simulink library "GOcontroll_Moduline_Target"  (R2018b)
settings: Solver=ode45  StartTime=0.0  StopTime=10.0  RelTol=1e-3  EnableMultiTasking=on
(part 3 of 3)

== system GOcontroll_Moduline_Target/Modules/Output Module ==
  Output Module (10 channel) : Subsystem  Tag=HANcoder_GOcontroll_Moduline_IV  mask(10 Channel Output Module){tsamp=0.1, ContrType=GOcontroll Moduline IV, moduleSlot=Moduleslot 1, C12freq=200 Hz, C1func=Disable (output disabled), C1peakDuty=1000, C1peakTime=500, C2func=Disable (output disabled), C2peakDuty=1000, C2peakTime=500, C34freq=200 Hz, C3func=Disable (output disabled), C3peakDuty=1000, C3peakTime=500, C4func=Disable (output disabled), C4peakDuty=1000, C4peakTime=500, C56freq=200 Hz, C5func=Disable (output disabled), C5peakDuty=1000, C5peakTime=500, C6func=Disable (output disabled), C6peakDuty=1000, C6peakTime=500, C78freq=200 Hz, C7func=Disable (output disabled), C7peakDuty=1000, C7peakTime=500, C8func=Disable (output disabled), C8peakDuty=1000, C8peakTime=500, C910freq=200 Hz, C9func=Disable (output disabled), C9peakDuty=1000, C9peakTime=500, C10func=Disable (output disabled), C10peakDuty=1000, C10peakTime=500}
      mask prompts: tsamp "Sample time"; ContrType "Controller type"; moduleSlot "Module slot"; C12freq "Frequency"; C1func "Channel 1 function"; C1peakDuty "Peak Duty-Cycle (0-1000)"; C1peakTime "Peak time (ms)"; C2func "Channel 2 function"; C2peakDuty "Peak Duty-Cycle (0-1000)"; C2peakTime "Peak time (ms)"; C34freq "Frequency"; C3func "Channel 3 function"; C3peakDuty "Peak Duty-Cycle (0-1000)"; C3peakTime "Peak time (ms)"; C4func "Channel 4 function"; C4peakDuty "Peak Duty-Cycle (0-1000)"; C4peakTime "Peak time (ms)"; C56freq "Frequency"; C5func "Channel 5 function"; C5peakDuty "Peak Duty-Cycle (0-1000)"; C5peakTime "Peak time (ms)"; C6func "Channel 6 function"; C6peakDuty "Peak Duty-Cycle (0-1000)"; C6peakTime "Peak time (ms)"; C78freq "Frequency"; C7func "Channel 7 function"; C7peakDuty "Peak Duty-Cycle (0-1000)"; C7peakTime "Peak time (ms)"; C8func "Channel 8 function"; C8peakDuty "Peak Duty-Cycle (0-1000)"; C8peakTime "Peak time (ms)"; C910freq "Frequency"; C9func "Channel 9 function"; C9peakDuty "Peak Duty-Cycle (0-1000)"; C9peakTime "Peak time (ms)"; C10func "Channel 10 function"; C10peakDuty "Peak Duty-Cycle (0-1000)"; C10peakTime "Peak time (ms)"
      mask help:
      | With this function block, you can configure each output of the 6 channel output module (202002xx). During initialization of the controller, the corresponding outputs of the module are set according the settings. During runtime, the value pushed into the block will control the outputs.
      |
      | Sample time:
      | Execution frequency from function block. For proper functioning of the output module, us a sampletime of 100 ms or lower.
      |
      | Module slot:
      | Sets the location of the module slot where the module is physically plugged into.
      |
      | Frequency:
      | In case a duty Cycle is used, select the frequency.
      |
      | Function select:
      | Select the desired output configuration for each channel
      mask init:
      | [moduleSlotInfoStr, connectorId, pin1Id, pin2Id, pin3Id, pin4Id, pin5Id, pin6Id, pin7Id, pin8Id, pin9Id, pin10Id] = sfcn_gocontroll_output_module_10_mcb(moduleSlot,ContrType,...
      | C12freq,C1func,C2func,C34freq,C3func,C4func,C56freq,C5func,C6func,C78freq,C7func,C8func,C910freq,C9func,C10func,...
      | C1peakDuty,C1peakTime,C2peakDuty,C2peakTime,C3peakDuty,C3peakTime,C4peakDuty,C4peakTime,C5peakDuty,C5peakTime,...
      | C6peakDuty,C6peakTime,C7peakDuty,C7peakTime,C8peakDuty,C8peakTime,C9peakDuty,C9peakTime,C10peakDuty,C10peakTime);
      settings: MoveFcn=%%drawLogos
      mask TypeOptions ContrType: GOcontroll Moduline IV | GOcontroll Moduline Mini | GOcontroll Moduline Display
      mask Callback ContrType:
      | msk = Simulink.Mask.get(gcb);
      | p = msk.Parameters;
      | 
      | func = get_param(gcb,'ContrType');
      | 
      | if(func == "GOcontroll Moduline IV")
      | p(3).TypeOptions = {'Moduleslot 1','Moduleslot 2','Moduleslot 3','Moduleslot 4',...
      |                     'Moduleslot 5','Moduleslot 6','Moduleslot 7','Moduleslot 8'};
      | elseif (func == "GOcontroll Moduline Mini")
      |  p(3).TypeOptions = {'Moduleslot 1','Moduleslot 2','Moduleslot 3','Moduleslot 4'};
      | 
      |  elseif (func == "GOcontroll Moduline Screen")
      |  p(3).TypeOptions = {'Moduleslot 1','Moduleslot 2'};
      | 
      | end
      mask TypeOptions moduleSlot: Moduleslot 1 | Moduleslot 2 | Moduleslot 3 | Moduleslot 4 | Moduleslot 5 | Moduleslot 6 | Moduleslot 7 | Moduleslot 8
      mask TypeOptions C12freq: 100 Hz | 200 Hz | 500 Hz | 1 kHz
      mask TypeOptions C1func: Disable (output disabled) | High side switch  dutycycle controlled (0 - 1000) | High side switch On - Off (0 - 1) | High side peak and hold (0 - 1000) | Frequency ouput 0 - 500 Hz (0 - 500)
      mask Callback C1func:
      | func = get_param(gcb,'C1func');
      | p=Simulink.Mask.get(gcb);
      | 
      | if( func == "High side peak and hold (0 - 1000)")
      | a=p.Parameters(6);
      | a.set('Visible','on');
      | a=p.Parameters(7);
      | a.set('Visible','on');
      | else
      | a=p.Parameters(6);
      | a.set('Visible','off');
      | a=p.Parameters(7);
      | a.set('Visible','off');
      | end
      mask TypeOptions C2func: Disable (output disabled) | High side switch  dutycycle controlled (0 - 1000) | High side switch On - Off (0 - 1) | High side peak and hold (0 - 1000) | Frequency ouput 0 - 500 Hz (0 - 500)
      mask Callback C2func:
      | func = get_param(gcb,'C2func');
      | p=Simulink.Mask.get(gcb);
      | 
      | if( func == "High side peak and hold (0 - 1000)")
      | a=p.Parameters(9);
      | a.set('Visible','on');
      | a=p.Parameters(10);
      | a.set('Visible','on');
      | else
      | a=p.Parameters(9);
      | a.set('Visible','off');
      | a=p.Parameters(10);
      | a.set('Visible','off');
      | end
      mask TypeOptions C34freq: 100 Hz | 200 Hz | 500 Hz | 1 kHz
      mask TypeOptions C3func: Disable (output disabled) | High side switch  dutycycle controlled (0 - 1000) | High side switch On - Off (0 - 1) | High side peak and hold (0 - 1000) | Frequency ouput 0 - 500 Hz (0 - 500)
      mask Callback C3func:
      | func = get_param(gcb,'C3func');
      | p=Simulink.Mask.get(gcb);
      | 
      | if( func == "High side peak and hold (0 - 1000)")
      | a=p.Parameters(13);
      | a.set('Visible','on');
      | a=p.Parameters(14);
      | a.set('Visible','on');
      | else
      | a=p.Parameters(13);
      | a.set('Visible','off');
      | a=p.Parameters(14);
      | a.set('Visible','off');
      | end
      mask TypeOptions C4func: Disable (output disabled) | High side switch  dutycycle controlled (0 - 1000) | High side switch On - Off (0 - 1) | High side peak and hold (0 - 1000) | Frequency ouput 0 - 500 Hz (0 - 500)
      mask Callback C4func:
      | func = get_param(gcb,'C4func');
      | p=Simulink.Mask.get(gcb);
      | 
      | if( func == "High side peak and hold (0 - 1000)")
      | a=p.Parameters(16);
      | a.set('Visible','on');
      | a=p.Parameters(17);
      | a.set('Visible','on');
      | else
      | a=p.Parameters(16);
      | a.set('Visible','off');
      | a=p.Parameters(17);
      | a.set('Visible','off');
      | end
      mask TypeOptions C56freq: 100 Hz | 200 Hz | 500 Hz | 1 kHz
      mask TypeOptions C5func: Disable (output disabled) | High side switch  dutycycle controlled (0 - 1000) | High side switch On - Off (0 - 1) | High side peak and hold (0 - 1000) | Frequency ouput 0 - 500 Hz (0 - 500)
      mask Callback C5func:
      | func = get_param(gcb,'C5func');
      | p=Simulink.Mask.get(gcb);
      | 
      | if( func == "High side peak and hold (0 - 1000)")
      | a=p.Parameters(20);
      | a.set('Visible','on');
      | a=p.Parameters(21);
      | a.set('Visible','on');
      | else
      | a=p.Parameters(20);
      | a.set('Visible','off');
      | a=p.Parameters(21);
      | a.set('Visible','off');
      | end
      mask TypeOptions C6func: Disable (output disabled) | High side switch  dutycycle controlled (0 - 1000) | High side switch On - Off (0 - 1) | High side peak and hold (0 - 1000) | Frequency ouput 0 - 500 Hz (0 - 500)
      mask Callback C6func:
      | func = get_param(gcb,'C6func');
      | p=Simulink.Mask.get(gcb);
      | 
      | if( func == "High side peak and hold (0 - 1000)")
      | a=p.Parameters(23);
      | a.set('Visible','on');
      | a=p.Parameters(24);
      | a.set('Visible','on');
      | else
      | a=p.Parameters(23);
      | a.set('Visible','off');
      | a=p.Parameters(24);
      | a.set('Visible','off');
      | end
      mask TypeOptions C78freq: 100 Hz | 200 Hz | 500 Hz | 1 kHz
      mask TypeOptions C7func: Disable (output disabled) | High side switch  dutycycle controlled (0 - 1000) | High side switch On - Off (0 - 1) | High side peak and hold (0 - 1000) | Frequency ouput 0 - 500 Hz (0 - 500)
      mask Callback C7func:
      | func = get_param(gcb,'C7func');
      | p=Simulink.Mask.get(gcb);
      | 
      | if( func == "High side peak and hold (0 - 1000)")
      | a=p.Parameters(27);
      | a.set('Visible','on');
      | a=p.Parameters(28);
      | a.set('Visible','on');
      | else
      | a=p.Parameters(27);
      | a.set('Visible','off');
      | a=p.Parameters(28);
      | a.set('Visible','off');
      | end
      mask TypeOptions C8func: Disable (output disabled) | High side switch  dutycycle controlled (0 - 1000) | High side switch On - Off (0 - 1) | High side peak and hold (0 - 1000) | Frequency ouput 0 - 500 Hz (0 - 500)
      mask Callback C8func:
      | func = get_param(gcb,'C8func');
      | p=Simulink.Mask.get(gcb);
      | 
      | if( func == "High side peak and hold (0 - 1000)")
      | a=p.Parameters(30);
      | a.set('Visible','on');
      | a=p.Parameters(31);
      | a.set('Visible','on');
      | else
      | a=p.Parameters(30);
      | a.set('Visible','off');
      | a=p.Parameters(31);
      | a.set('Visible','off');
      | end
      mask TypeOptions C910freq: 100 Hz | 200 Hz | 500 Hz | 1 kHz
      mask TypeOptions C9func: Disable (output disabled) | High side switch  dutycycle controlled (0 - 1000) | High side switch On - Off (0 - 1) | High side peak and hold (0 - 1000) | Frequency ouput 0 - 500 Hz (0 - 500)
      mask Callback C9func:
      | func = get_param(gcb,'C9func');
      | p=Simulink.Mask.get(gcb);
      | 
      | if( func == "High side peak and hold (0 - 1000)")
      | a=p.Parameters(34);
      | a.set('Visible','on');
      | a=p.Parameters(35);
      | a.set('Visible','on');
      | else
      | a=p.Parameters(34);
      | a.set('Visible','off');
      | a=p.Parameters(35);
      | a.set('Visible','off');
      | end
      mask TypeOptions C10func: Disable (output disabled) | High side switch  dutycycle controlled (0 - 1000) | High side switch On - Off (0 - 1) | High side peak and hold (0 - 1000) | Frequency ouput 0 - 500 Hz (0 - 500)
      mask Callback C10func:
      | func = get_param(gcb,'C10func');
      | p=Simulink.Mask.get(gcb);
      | 
      | if( func == "High side peak and hold (0 - 1000)")
      | a=p.Parameters(37);
      | a.set('Visible','on');
      | a=p.Parameters(38);
      | a.set('Visible','on');
      | else
      | a=p.Parameters(37);
      | a.set('Visible','off');
      | a=p.Parameters(38);
      | a.set('Visible','off');
      | end
      mask DialogControl Container9 Prompt: Output 1 and 2
      mask DialogControl Container12 Prompt: Output 3 and 4
      mask DialogControl Container13 Prompt: Output 5 and 6
      mask DialogControl Container14 Prompt: Output 7 and 8
      mask DialogControl Container15 Prompt: Output 9 and 10
      mask Display:
      | fprintf('10 Channel Output Module\n%s\n\n Controller Connector: %s', moduleSlotInfoStr,connectorId);%%connectorId
      | port_label('input', 1, pin1Id);
      | port_label('input', 2, pin2Id);
      | port_label('input', 3, pin3Id);
      | port_label('input', 4, pin4Id);
      | port_label('input', 5, pin5Id);
      | port_label('input', 6, pin6Id);
      | port_label('input', 7, pin3Id);
      | port_label('input', 8, pin4Id);
      | port_label('input', 9, pin5Id);
      | port_label('input', 10, pin6Id);
      | text(2, 6, ert_linux_target_version());
  Output Module (6 channel) : Subsystem  Tag=HANcoder_GOcontroll_Moduline_IV  mask(6 Channel Output Module){tsamp=0.1, ContrType=GOcontroll Moduline IV, moduleSlot=Moduleslot 1, C12freq=200 Hz, C1func=Disable (output disabled), C1cur=4000, C1peakCurrent=1000, C1peakTime=500, C2func=Disable (output disabled), C2cur=4000, C2peakCurrent=1000, C2peakTime=500, C34freq=200 Hz, C3func=Disable (output disabled), C3cur=4000, C3peakCurrent=1000, C3peakTime=500, C4func=Disable (output disabled), C4cur=4000, C4peakCurrent=1000, C4peakTime=500, C56freq=200 Hz, C5func=Disable (output disabled), C5cur=4000, C5peakCurrent=1000, C5peakTime=500, C6func=Disable (output disabled), C6cur=4000, C6peakCurrent=1000, C6peakTime=500}
      mask prompts: tsamp "Sample time"; ContrType "Controller Type"; moduleSlot "Module slot"; C12freq "Frequency"; C1func "Channel 1 function"; C1cur "Channel 1 Imax [mA]"; C1peakCurrent "Peak Current [mA]"; C1peakTime "Peak time [ms]"; C2func "Channel 2 function"; C2cur "Channel 2 Imax [mA]"; C2peakCurrent "Peak Current [mA]"; C2peakTime "Peak time [ms]"; C34freq "Frequency"; C3func "Channel 3 function"; C3cur "Channel 3 Imax [mA]"; C3peakCurrent "Peak Current [mA]"; C3peakTime "Peak time [ms]"; C4func "Channel 4 function"; C4cur "Channel 4 Imax [mA]"; C4peakCurrent "Peak Current [mA]"; C4peakTime "Peak time [ms]"; C56freq "Frequency"; C5func "Channel 5 function"; C5cur "Channel 5 Imax [mA]"; C5peakCurrent "Peak Current [mA]"; C5peakTime "Peak time [ms]"; C6func "Channel 6 function"; C6cur "Channel 6 Imax [mA]"; C6peakCurrent "Peak Current [mA]"; C6peakTime "Peak time [ms]"
      mask help:
      | With this function block, you can configure each output of the 6 channel output module (202002xx). During initialization of the controller, the corresponding outputs of the module are set according the settings. During runtime, the value pushed into the block will control the outputs.
      |
      | Sample time:
      | Execution frequency from function block. For proper functioning of the output module, us a sampletime of 100 ms or lower.
      |
      | Module slot:
      | Sets the location of the module slot where the module is physically plugged into.
      |
      | Frequency:
      | In case a duty Cycle is used, select the frequency.
      |
      | Function select:
      | Select the desired output configuration for each channel
      mask init:
      | [moduleSlotInfoStr, connectorId, pin1Id, pin2Id, pin3Id, pin4Id, pin5Id, pin6Id] = sfcn_gocontroll_output_module_mcb(moduleSlot,ContrType,...
      | C12freq,C1func,C2func,C34freq,C3func,C4func,C56freq,C5func,C6func,C1cur,C2cur,C3cur,C4cur,C5cur,C6cur,...
      | C1peakCurrent,C1peakTime,C2peakCurrent,C2peakTime,C3peakCurrent,C3peakTime,C4peakCurrent,C4peakTime,C5peakCurrent,C5peakTime,C6peakCurrent,C6peakTime);
      settings: MoveFcn=%%drawLogos
      mask TypeOptions ContrType: GOcontroll Moduline IV | GOcontroll Moduline Mini | GOcontroll Moduline Display
      mask Callback ContrType:
      | msk = Simulink.Mask.get(gcb);
      | p = msk.Parameters;
      | 
      | func = get_param(gcb,'ContrType');
      | 
      | if(func == "GOcontroll Moduline IV")
      | p(3).TypeOptions = {'Moduleslot 1','Moduleslot 2','Moduleslot 3','Moduleslot 4',...
      |                     'Moduleslot 5','Moduleslot 6','Moduleslot 7','Moduleslot 8'};
      | elseif(func == "GOcontroll Moduline Mini")
      |  p(3).TypeOptions = {'Moduleslot 1','Moduleslot 2','Moduleslot 3','Moduleslot 4'};
      | 
      | elseif (func == "GOcontroll Moduline Screen")
      |  p(3).TypeOptions = {'Moduleslot 1','Moduleslot 2'};
      | end
      mask TypeOptions moduleSlot: Moduleslot 1 | Moduleslot 2 | Moduleslot 3 | Moduleslot 4 | Moduleslot 5 | Moduleslot 6 | Moduleslot 7 | Moduleslot 8
      mask TypeOptions C12freq: 100 Hz | 200 Hz | 500 Hz | 1 kHz | 2 kHz | 5 kHz | 10 kHz
      mask TypeOptions C1func: Disable (output disabled) | Half Bridge dutycycle controlled (0 - 1000) | Low side switch  dutycycle controlled (0 - 1000) | High side switch  dutycycle controlled (0 - 1000) | Low side switch On - Off (0 - 1) | High side switch On - Off (0 - 1) | Peak and hold current mode (Half Bridge) | Frequency output 0 - 500 Hz (0-500)
      mask Callback C1func:
      | func = get_param(gcb,'C1func');
      | p=Simulink.Mask.get(gcb);
      | 
      | if( func == "Peak and hold current mode (Half Bridge)")
      | a=p.Parameters(7);
      | a.set('Visible','on');
      | a=p.Parameters(8);
      | a.set('Visible','on');
      | else
      | a=p.Parameters(7);
      | a.set('Visible','off');
      | a=p.Parameters(8);
      | a.set('Visible','off');
      | end
      | 
      | if( func == "Disable (output disabled)")
      | a=p.Parameters(6);
      | a.set('Enabled','off');
      | else
      | a=p.Parameters(6);
      | a.set('Enabled','on');
      | end
      mask TypeOptions C2func: Disable (output disabled) | Half Bridge dutycycle controlled (0 - 1000) | Low side switch  dutycycle controlled (0 - 1000) | High side switch  dutycycle controlled (0 - 1000) | Low side switch On - Off (0 - 1) | High side switch On - Off (0 - 1) | Peak and hold current mode (Half Bridge) | Frequency output 0 - 500 Hz (0-500)
      mask Callback C2func:
      | func = get_param(gcb,'C2func');
      | p=Simulink.Mask.get(gcb);
      | 
      | if( func == "Peak and hold current mode (Half Bridge)")
      | a=p.Parameters(11);
      | a.set('Visible','on');
      | a=p.Parameters(12);
      | a.set('Visible','on');
      | else
      | a=p.Parameters(11);
      | a.set('Visible','off');
      | a=p.Parameters(12);
      | a.set('Visible','off');
      | end
      | 
      | if( func == "Disable (output disabled)")
      | a=p.Parameters(10);
      | a.set('Enabled','off');
      | else
      | a=p.Parameters(10);
      | a.set('Enabled','on');
      | end
      mask TypeOptions C34freq: 100 Hz | 200 Hz | 500 Hz | 1 kHz | 2 kHz | 5 kHz | 10 kHz
      mask TypeOptions C3func: Disable (output disabled) | Half Bridge dutycycle controlled (0 - 1000) | Low side switch  dutycycle controlled (0 - 1000) | High side switch  dutycycle controlled (0 - 1000) | Low side switch On - Off (0 - 1) | High side switch On - Off (0 - 1) | Peak and hold current mode (Half Bridge) | Frequency output 0 - 500 Hz (0-500)
      mask Callback C3func:
      | func = get_param(gcb,'C3func');
      | p=Simulink.Mask.get(gcb);
      | 
      | if( func == "Peak and hold current mode (Half Bridge)")
      | a=p.Parameters(16);
      | a.set('Visible','on');
      | a=p.Parameters(17);
      | a.set('Visible','on');
      | else
      | a=p.Parameters(16);
      | a.set('Visible','off');
      | a=p.Parameters(17);
      | a.set('Visible','off');
      | end
      | 
      | if( func == "Disable (output disabled)")
      | a=p.Parameters(15);
      | a.set('Enabled','off');
      | else
      | a=p.Parameters(15);
      | a.set('Enabled','on');
      | end
      mask TypeOptions C4func: Disable (output disabled) | Half Bridge dutycycle controlled (0 - 1000) | Low side switch  dutycycle controlled (0 - 1000) | High side switch  dutycycle controlled (0 - 1000) | Low side switch On - Off (0 - 1) | High side switch On - Off (0 - 1) | Peak and hold current mode (Half Bridge) | Frequency output 0 - 500 Hz (0-500)
      mask Callback C4func:
      | func = get_param(gcb,'C4func');
      | p=Simulink.Mask.get(gcb);
      | 
      | if( func == "Peak and hold current mode (Half Bridge)")
      | a=p.Parameters(20);
      | a.set('Visible','on');
      | a=p.Parameters(21);
      | a.set('Visible','on');
      | else
      | a=p.Parameters(20);
      | a.set('Visible','off');
      | a=p.Parameters(21);
      | a.set('Visible','off');
      | end
      | 
      | if( func == "Disable (output disabled)")
      | a=p.Parameters(19);
      | a.set('Enabled','off');
      | else
      | a=p.Parameters(19);
      | a.set('Enabled','on');
      | end
      mask TypeOptions C56freq: 100 Hz | 200 Hz | 500 Hz | 1 kHz | 2 kHz | 5 kHz | 10 kHz
      mask TypeOptions C5func: Disable (output disabled) | Half Bridge dutycycle controlled (0 - 1000) | Low side switch  dutycycle controlled (0 - 1000) | High side switch  dutycycle controlled (0 - 1000) | Low side switch On - Off (0 - 1) | High side switch On - Off (0 - 1) | Peak and hold current mode (Half Bridge) | Frequency output 0 - 500 Hz (0-500)
      mask Callback C5func:
      | func = get_param(gcb,'C5func');
      | p=Simulink.Mask.get(gcb);
      | 
      | if( func == "Peak and hold current mode (Half Bridge)")
      | a=p.Parameters(25);
      | a.set('Visible','on');
      | a=p.Parameters(26);
      | a.set('Visible','on');
      | else
      | a=p.Parameters(25);
      | a.set('Visible','off');
      | a=p.Parameters(26);
      | a.set('Visible','off');
      | end
      | 
      | if( func == "Disable (output disabled)")
      | a=p.Parameters(24);
      | a.set('Enabled','off');
      | else
      | a=p.Parameters(24);
      | a.set('Enabled','on');
      | end
      mask TypeOptions C6func: Disable (output disabled) | Half Bridge dutycycle controlled (0 - 1000) | Low side switch  dutycycle controlled (0 - 1000) | High side switch  dutycycle controlled (0 - 1000) | Low side switch On - Off (0 - 1) | High side switch On - Off (0 - 1) | Peak and hold current mode (Half Bridge) | Frequency output 0 - 500 Hz (0-500)
      mask Callback C6func:
      | func = get_param(gcb,'C6func');
      | p=Simulink.Mask.get(gcb);
      | 
      | if( func == "Peak and hold current mode (Half Bridge)")
      | a=p.Parameters(29);
      | a.set('Visible','on');
      | a=p.Parameters(30);
      | a.set('Visible','on');
      | else
      | a=p.Parameters(29);
      | a.set('Visible','off');
      | a=p.Parameters(30);
      | a.set('Visible','off');
      | end
      | 
      | if( func == "Disable (output disabled)")
      | a=p.Parameters(28);
      | a.set('Enabled','off');
      | else
      | a=p.Parameters(28);
      | a.set('Enabled','on');
      | end
      mask DialogControl Container9 Prompt: Output 1 and 2
      mask DialogControl Container12 Prompt: Output 3 and 4
      mask DialogControl Container13 Prompt: Output 5 and 6
      mask Display:
      | fprintf('6 Channel Output Module\n%s\n\n Controller Connector: %s', moduleSlotInfoStr,connectorId);%%connectorId
      | port_label('input', 1, pin1Id);
      | port_label('input', 2, pin2Id);
      | port_label('input', 3, pin3Id);
      | port_label('input', 4, pin4Id);
      | port_label('input', 5, pin5Id);
      | port_label('input', 6, pin6Id);
      | text(2, 6, ert_linux_target_version());
  Output Module Monitor (6 channel) : Subsystem  Tag=HANcoder_GOcontroll_Moduline_IV  mask(Output Module Monitor){tsamp=0.1, ContrType=GOcontroll Moduline IV, moduleSlot=Moduleslot 1}
      mask prompts: tsamp "Sample time"; ContrType "Controller Type"; moduleSlot "Module Slot"
      mask help:
      | With this function block, you can read parameters from the specified 6 channel output module (202002xx). The block will provide some information about the module such as:
      |
      | Module temperature:
      | The temperature in degrees from the output module.
      |
      | Module ground shift
      | In case the ground connection of the module is poor, the power ground is shifted. The value gives the ground difference in mV and schould be beneath 50 mV
      |
      | Channel current
      | The current from each channel is measured and given in mA. If the ouput is configured as high side, the result will be positive. If the ouput is configured as low side, the value will be negative
      mask init:
      | [moduleSlotInfoStr, connectorId, pin1Id, pin2Id, pin3Id, pin4Id, pin5Id, pin6Id] = sfcn_gocontroll_output_module_monitor_mcb(moduleSlot,ContrType);
      settings: MoveFcn=%%drawLogos
      mask TypeOptions ContrType: GOcontroll Moduline IV | GOcontroll Moduline Mini | GOcontroll Moduline Display
      mask Callback ContrType:
      | msk = Simulink.Mask.get(gcb);
      | p = msk.Parameters;
      | 
      | func = get_param(gcb,'ContrType');
      | 
      | if(func == "GOcontroll Moduline IV")
      | p(3).TypeOptions = {'Moduleslot 1','Moduleslot 2','Moduleslot 3','Moduleslot 4',...
      |                     'Moduleslot 5','Moduleslot 6','Moduleslot 7','Moduleslot 8'};
      | 
      | elseif (func == "GOcontroll Moduline Mini")
      |  p(3).TypeOptions = {'Moduleslot 1','Moduleslot 2','Moduleslot 3','Moduleslot 4'};
      | 
      | elseif (func == "GOcontroll Moduline Screen")
      |  p(3).TypeOptions = {'Moduleslot 1','Moduleslot 2'};
      | 
      | end
      mask TypeOptions moduleSlot: Moduleslot 1 | Moduleslot 2 | Moduleslot 3 | Moduleslot 4 | Moduleslot 5 | Moduleslot 6 | Moduleslot 7 | Moduleslot 8
      mask Display:
      | fprintf('6 Channel Output Module Monitor\n%s\n\n Controller Connector: %s', moduleSlotInfoStr,connectorId);
      | port_label('output', 1, 'Temperature');
      | port_label('output', 2, 'Groundshift');
      | port_label('output', 3, 'Status');
      | port_label('output', 4, pin1Id);
      | port_label('output', 5, pin2Id);
      | port_label('output', 6, pin3Id);
      | port_label('output', 7, pin4Id);
      | port_label('output', 8, pin5Id);
      | port_label('output', 9, pin6Id);
      | text(2, 6, ert_linux_target_version());

== system GOcontroll_Moduline_Target/Network/MQTT ==

== system GOcontroll_Moduline_Target/Network/UDP ==
  Configure UDP socket : Subsystem  mask(Configure UDP socket){port=9001, ip='0.0.0.0', broadcast=on, tsamp=0.01}
      mask prompts: port "The port on which to listen"; ip "The ip on which to listen"; broadcast "Allow broadcasting of send messages"; tsamp "Sample time"
      mask help: Block to configure a UDP connection
      mask init:
      | if broadcast == 0
      |     broadcastStr = "Not broadcasting";
      | else
      |     broadcastStr = "Broadcasting";
      | end
      mask Help:
      | Setting the ip to 0.0.0.0 makes the controller accept messages on all interfaces.
      | Set it to the ip of a specific interface to limit this.
      | 
      | Allowing broadcasting enables you to send messages to a full range of ip addresses, for example:
      | 192.168.255.255 sends messages to 192.168.1.1, 192.168.2.1 ... 192.168.1.2, 192.168.1.3...
      mask Display:
      | fprintf('Configure UDP socket\n IP: %s\nPort: %d\n%s',ip,port,broadcastStr);
      | text(2, 6, ert_linux_target_version());
  UDP Send : M-S-Function  FunctionName=sfcn_UDPSend  Parameters=tsamp,port,ip,id,input_type  mask(UDP send){input_type=off, id=0, ip='0.0.0.0', port=0, tsamp=1}
      mask prompts: input_type "Use input for ID"; id "Message ID"; ip "The IP address to send to"; port "The port to send to"; tsamp "Sample time"
      mask help:
      | Send a UDP packet
      |
      | Inputs:
      | ID:
      | The message identifier, start from 0 going up with no gaps
      |
      | Message:
      | A [uint8] to send with the UDP protocol.
      mask Callback input_type:
      | type = get_param(gcb, 'input_type');
      | if strcmp(type, 'on')
      |     set_param(gcb, 'MaskVisibilities',{'on','off','on','on','on'});
      | else
      |     set_param(gcb, 'MaskVisibilities',{'on','on' ,'on','on','on'});
      | end
      | 
      | clear type
      mask Display:
      | if input_type
      |     fprintf('UDP Send\nIP: %s\nPort: %d',ip,port);
      |     port_label('input', 1, 'ID');
      |     port_label('input', 2, 'message');
      | else
      |     fprintf('UDP Send\nIP: %s\nPort: %d\n ID: %d',ip,port,id);
      |     port_label('input', 1, 'message');
      | end
      | text(2, 6, ert_linux_target_version());
  UDP Send old : Subsystem  mask(UDP send){input_type=off, id=0, ip='255.255.255.255', port=9001, tsamp=0.01}
      mask prompts: input_type "Use input for ID"; id "Message ID"; ip "The IP address to send to"; port "The port to send to"; tsamp "Sample time"
      mask help:
      | Send a UDP packet
      |
      | Inputs:
      | ID:
      | The message identifier, start from 0 going up with no gaps
      |
      | Message:
      | A [uint8] to send with the UDP protocol.
      mask init:
      | if input_type
      |     if getSimulinkBlockHandle([gcb '/Gnd']) > 0
      |         %Get the position of the ground block
      |         thisPosition = get_param ([gcb, '/Gnd'], 'Position');
      |         % Remove the ground block
      |         delete_block ([gcb, '/Gnd']);
      |         % Add a input block
      |         add_block ('built-in/Inport', [gcb, '/ID']);
      |         %Allign the new input block to be placed at the position of the
      |         % removed ground
      |         set_param ([gcb, '/ID'], 'Position', thisPosition);
      |         set_param ([gcb, '/ID'], 'Port', '1');
      |         clear thisPosition
      |     end
      | else
      |     if getSimulinkBlockHandle([gcb '/ID']) > 0
      |         % Get the position of the input block
      |         thisPosition = get_param ([gcb, '/ID'], 'Position');
      |         % Remove the input block
      |         delete_block ([gcb, '/ID']);
      |         % Add a ground block
      |         add_block ('built-in/Ground', [gcb, '/Gnd']);
      |         % Allign the new ground block to be placed at the position of the
      |         % removed input
      |         set_param ([gcb, '/Gnd'], 'Position', thisPosition);
      |         clear thisPosition
      |     end
      | end
      | 
      | sfcn_UDPSend_mcb(port,ip,id,input_type);
      mask Callback input_type:
      | type = get_param(gcb, 'input_type');
      | if strcmp(type, 'on')
      |     set_param(gcb, 'MaskVisibilities',{'on','off','on','on','on'});
      | else
      |     set_param(gcb, 'MaskVisibilities',{'on','on' ,'on','on','on'});
      | end
      | 
      | clear type
      mask Display:
      | if input_type
      |     fprintf('UDP Send\nIP: %s\nPort: %d',ip,port);
      | else
      |     fprintf('UDP Send\nIP: %s\nPort: %d\n ID: %d',ip,port,id);
      | end
      | text(2, 6, ert_linux_target_version());
  UDP receive : M-S-Function  FunctionName=sfcn_UDPReceive  Parameters=tsamp,id,buff_len,input_type  mask(UDP receive){input_type=off, id=0, buff_len=1, tsamp=1}
      mask prompts: input_type "Use input for ID"; id "Message ID/Number of buffers"; buff_len "Buffer size"; tsamp "Sample time"
      mask help:
      | Receive UDP messages
      |
      | parameters:
      |
      | Use input for ID
      | Configure the ID with an input port instead of a parameter
      | Usecase is for example a for iter subsystem to read out multiple IDs
      |
      | ID/Number of buffers
      | ID byte of the message
      | The number of buffers allocated is the highest ID in the model + 1 so build it up from 0
      | When the ID is configured as an input and not the parameter this value will still determine the number of receive buffers.
      |
      | Buffer size
      | The size of the message that will be received in this block in number of bytes
      |
      | Output:
      |
      | 1. newMessage
      | Flag to tell if a new message arrived
      |
      | 2. Message
      | the Message in the form of [uint8;buffsize]
      mask Display:
      | if input_type
      |     fprintf('UDP Receive');
      | else
      |     fprintf('UDP Receive\nID: %d',id);
      | end
      | text(2, 6, ert_linux_target_version());
      | port_label('output', 1, 'new message');
      | port_label('output', 2, 'message');
      | if input_type
      |     port_label('input', 1, 'ID');
      | end
  UDP receive old : Subsystem  mask(UDP receive){input_type=off, id=1, buff_len=1, tsamp=0.01}
      mask prompts: input_type "Use input for ID"; id "Message ID/Number of buffers"; buff_len "Buffer size"; tsamp "Sample time"
      mask help:
      | Receive UDP messages
      |
      | parameters:
      |
      | Use input for ID
      | Configure the ID with an input port instead of a parameter
      | Usecase is for example a for iter subsystem to read out multiple IDs
      |
      | ID/Number of buffers
      | ID byte of the message
      | The number of buffers allocated is the highest ID in the model + 1 so build it up from 0
      | When the ID is configured as an input and not the parameter this value will still determine the number of receive buffers.
      |
      | Buffer size
      | The size of the message that will be received in this block in number of bytes
      |
      | Output:
      |
      | 1. newMessage
      | Flag to tell if a new message arrived
      |
      | 2. Message
      | the Message in the form of [uint8;buffsize]
      mask init:
      | % if input_type
      | %     if getSimulinkBlockHandle([gcb '/Gnd']) > 0
      | %         %Get the position of the ground block
      | %         thisPosition = get_param ([gcb, '/Gnd'], 'Position');
      | %         % Remove the ground block
      | %         delete_block ([gcb, '/Gnd']);
      | %         % Add a input block
      | %         add_block ('built-in/Inport', [gcb, '/ID']);
      | %         %Allign the new input block to be placed at the position of the
      | %         % removed ground
      | %         set_param ([gcb, '/ID'], 'Position', thisPosition);
      | %     end
      | % else
      | %     if getSimulinkBlockHandle([gcb '/ID']) > 0
      | %         % Get the position of the input block
      | %         thisPosition = get_param ([gcb, '/ID'], 'Position');
      | %         % Remove the input block
      | %         delete_block ([gcb, '/ID']);
      | %         % Add a ground block
      | %         add_block ('built-in/Ground', [gcb, '/Gnd']);
      | %         % Allign the new ground block to be placed at the position of the
      | %         % removed input
      | %         set_param ([gcb, '/Gnd'], 'Position', thisPosition);
      | %     end
      | % end
      | % 
      | % sfcn_UDPReceive_mcb(id, buff_len, input_type);
      mask Callback input_type:
      | % type = get_param(gcb, 'input_type');
      | % messageID = Simulink.Mask.get(gcb);
      | % IDParam = messageID(1);
      | % if strcmp(type, 'on')
      | %     IDParam.set('Prompt','Number of receive buffers');
      | %     %set_param(gcb, 'MaskVisibilities',{'on','off','on','on'});
      | % else
      | %     IDParam.set('Prompt','Message ID');
      | %     %set_param(gcb, 'MaskVisibilities',{'on','on','on','on'});
      | % end
      | %
      | % clear type messageID IDParam
      mask Display:
      | if input_type
      |     fprintf('UDP Receive');
      | else
      |     fprintf('UDP Receive\nID: %d',id);
      | end
      | text(2, 6, ert_linux_target_version());

== system GOcontroll_Moduline_Target/Supply control/Controller Active ==
  In1 : Inport
  Level-2 M-file S-Function : M-S-Function  FunctionName=sfcn_gocontroll_controller_active  Parameters=tsamp
  wires:
  In1/1 -> Level-2 M-file S-Function/1

== system GOcontroll_Moduline_Target/Supply control/K15 Voltage ==
  Level-2 M-file S-Function : M-S-Function  FunctionName=sfcn_gocontroll_k15_voltage  Parameters=tsamp, k15pin
  Out1 : Outport
  wires:
  Level-2 M-file S-Function/1 -> Out1/1

== system GOcontroll_Moduline_Target/Supply control/K30 Voltage ==
  Level-2 M-file S-Function : M-S-Function  FunctionName=sfcn_gocontroll_k30_voltage  Parameters=tsamp
  Out1 : Outport
  wires:
  Level-2 M-file S-Function/1 -> Out1/1

== system GOcontroll_Moduline_Target/System/Build Settings ==

== system GOcontroll_Moduline_Target/System/CPU ==
  Level-2 M-file S-Function : M-S-Function  FunctionName=sfcn_gocontroll_cpu_temperature  Parameters=tsamp
  Out1 : Outport
  wires:
  Level-2 M-file S-Function/1 -> Out1/1

== system GOcontroll_Moduline_Target/System/License Key ==
  Level-2 M-file S-Function : M-S-Function  FunctionName=sfcn_license_key  Parameters=tsamp, key, iv, license, check_file

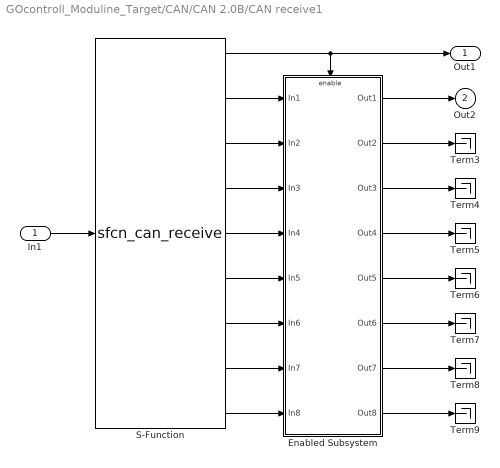
== system GOcontroll_Moduline_Target/CAN/CAN 2.0B/CAN receive1 ==
  In1 : Inport
  Enabled Subsystem : Subsystem  TreatAsAtomicUnit=on
  S-Function : M-S-Function  FunctionName=sfcn_can_receive  Parameters=tsamp, canBus, outputNumber, dataType, byteOrder
  Term{3..9} (7 alike) : Terminator
  Out1 : Outport
  Out2 : Outport  Port=2
  wires:
  In1/1 -> S-Function/1
  S-Function/1 -> Enabled Subsystem/Enable, Out1/1
  S-Function/6 -> Enabled Subsystem/5(In5)
  S-Function/5 -> Enabled Subsystem/4(In4)
  S-Function/9 -> Enabled Subsystem/8(In8)
  S-Function/2 -> Enabled Subsystem/1(In1)
  S-Function/3 -> Enabled Subsystem/2(In2)
  S-Function/4 -> Enabled Subsystem/3(In3)
  S-Function/8 -> Enabled Subsystem/7(In7)
  S-Function/7 -> Enabled Subsystem/6(In6)
  Enabled Subsystem/1(Out1) -> Out2/1
  Enabled Subsystem/2(Out2) -> Term3/1
  Enabled Subsystem/3(Out3) -> Term4/1
  Enabled Subsystem/4(Out4) -> Term5/1
  Enabled Subsystem/5(Out5) -> Term6/1
  Enabled Subsystem/6(Out6) -> Term7/1
  Enabled Subsystem/7(Out7) -> Term8/1
  Enabled Subsystem/8(Out8) -> Term9/1

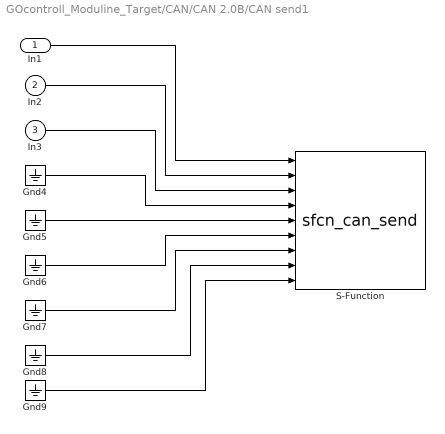
== system GOcontroll_Moduline_Target/CAN/CAN 2.0B/CAN send1 ==
  In1 : Inport
  In2 : Inport  Port=2
  In3 : Inport  Port=3
  Gnd{4..9} (6 alike) : Ground
  S-Function : M-S-Function  FunctionName=sfcn_can_send  Parameters=tsamp, canBus, frameType, inputNumber, dataType, byteOrder,RTR
  wires:
  In1/1 -> S-Function/1
  In2/1 -> S-Function/2
  In3/1 -> S-Function/3
  Gnd4/1 -> S-Function/4
  Gnd5/1 -> S-Function/5
  Gnd6/1 -> S-Function/6
  Gnd7/1 -> S-Function/7
  Gnd8/1 -> S-Function/8
  Gnd9/1 -> S-Function/9

== system GOcontroll_Moduline_Target/Memory store/Diagnostic to memory/Delete all codes for one group ==
  Trigger : TriggerPort  VariantControl=Variant  PortDimensions=1
  Level-2 M-file S-Function : M-S-Function  FunctionName=sfcn_memory_diagnostic_delete_code  Parameters=tsamp,diagType

== system GOcontroll_Moduline_Target/Memory store/Diagnostic to memory/Number of stored diagnostic codes ==
  Level-2 M-file S-Function : M-S-Function  FunctionName=sfcn_memory_diagnostic_nrcodes_read  Parameters=tsamp,diagType
  Out1 : Outport
  wires:
  Level-2 M-file S-Function/1 -> Out1/1

== system GOcontroll_Moduline_Target/Memory store/Diagnostic to memory/Read diagnostic code ==
  In1 : Inport
  In2 : Inport  Port=2
  Level-2 M-file S-Function : M-S-Function  FunctionName=sfcn_memory_diagnostic_read_code  Parameters=tsamp
  Out1 : Outport
  wires:
  Level-2 M-file S-Function/1 -> Out1/1
  In1/1 -> Level-2 M-file S-Function/1
  In2/1 -> Level-2 M-file S-Function/2

== system GOcontroll_Moduline_Target/Memory store/Diagnostic to memory/Store diagnostic code ==
  In1 : Inport
  Trigger : TriggerPort  VariantControl=Variant  PortDimensions=1
  Level-2 M-file S-Function : M-S-Function  FunctionName=sfcn_memory_diagnostic_write_code  Parameters=tsamp,diagType
  wires:
  In1/1 -> Level-2 M-file S-Function/1

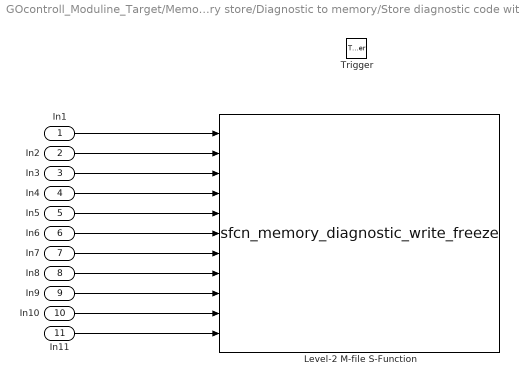
== system GOcontroll_Moduline_Target/Memory store/Diagnostic to memory/Store diagnostic code with freeze frame ==
  In1 : Inport
  In2 : Inport  Port=2
  In3 : Inport  Port=3
  In4 : Inport  Port=4
  In5 : Inport  Port=5
  In6 : Inport  Port=6
  In7 : Inport  Port=7
  In8 : Inport  Port=8
  In9 : Inport  Port=9
  In10 : Inport  Port=10
  In11 : Inport  Port=11
  Trigger : TriggerPort  VariantControl=Variant  PortDimensions=1
  Level-2 M-file S-Function : M-S-Function  FunctionName=sfcn_memory_diagnostic_write_freeze  Parameters=tsamp,diagType,FreezeParam1,FreezeParam2,FreezeParam3,FreezeParam4,FreezeParam5,FreezeParam6,FreezeParam7,FreezeParam8,FreezeParam9,FreezeParam10
  wires:
  In1/1 -> Level-2 M-file S-Function/1
  In3/1 -> Level-2 M-file S-Function/3
  In2/1 -> Level-2 M-file S-Function/2
  In4/1 -> Level-2 M-file S-Function/4
  In7/1 -> Level-2 M-file S-Function/7
  In6/1 -> Level-2 M-file S-Function/6
  In8/1 -> Level-2 M-file S-Function/8
  In5/1 -> Level-2 M-file S-Function/5
  In9/1 -> Level-2 M-file S-Function/9
  In11/1 -> Level-2 M-file S-Function/11
  In10/1 -> Level-2 M-file S-Function/10

== system GOcontroll_Moduline_Target/Memory store/Variable to memory/Memory read ==
  Level-2 M-file S-Function : M-S-Function  FunctionName=sfcn_memory_emulation_read  Parameters=tsamp,key,memRead,memType
  Out1 : Outport
  wires:
  Level-2 M-file S-Function/1 -> Out1/1

== system GOcontroll_Moduline_Target/Memory store/Variable to memory/Memory write ==
  In1 : Inport
  Level-2 M-file S-Function : M-S-Function  FunctionName=sfcn_memory_emulation_write  Parameters=tsamp,key,memType
  wires:
  In1/1 -> Level-2 M-file S-Function/1

== system GOcontroll_Moduline_Target/Modules/Bridge Module/Bridge Module ==
  In1 : Inport
  In2 : Inport  Port=2
  Level-2 M-file S-Function : M-S-Function  FunctionName=sfcn_gocontroll_bridge_module  Parameters=tsamp, moduleSlot,C1func,C1freq,C2func,C2freq
  wires:
  In2/1 -> Level-2 M-file S-Function/2
  In1/1 -> Level-2 M-file S-Function/1

== system GOcontroll_Moduline_Target/Modules/Bridge Module/Bridge Module Monitor ==
  Level-2 M-file S-Function : M-S-Function  FunctionName=sfcn_gocontroll_bridge_module_monitor  Parameters=tsamp, moduleSlot
  Out1 : Outport
  Out2 : Outport  Port=2
  Out3 : Outport  Port=3
  Out4 : Outport  Port=4
  wires:
  Level-2 M-file S-Function/4 -> Out4/1
  Level-2 M-file S-Function/3 -> Out3/1
  Level-2 M-file S-Function/2 -> Out2/1
  Level-2 M-file S-Function/1 -> Out1/1

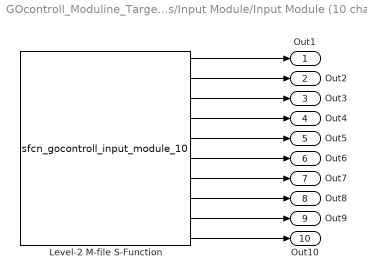
== system GOcontroll_Moduline_Target/Modules/Input Module/Input Module (10 channel) ==
  Level-2 M-file S-Function : M-S-Function  FunctionName=sfcn_gocontroll_input_module_10  Parameters=tsamp, moduleSlot,C1func,C1pu,C1pd,C2func,C2pu,C2pd,C3func,C3pu,C3pd,C4func,C4pu,C4pd,C5func,C5pu,C5pd,C6func,C6pu,C6pd,C7func,C7pu,C7pd,C8func,C8pu,C8pd,C9func,C9pu,C9pd,C10func,C10pu,C10pd,SensSup1
  Out1 : Outport
  Out2 : Outport  Port=2
  Out3 : Outport  Port=3
  Out4 : Outport  Port=4
  Out5 : Outport  Port=5
  Out6 : Outport  Port=6
  Out7 : Outport  Port=7
  Out8 : Outport  Port=8
  Out9 : Outport  Port=9
  Out10 : Outport  Port=10
  wires:
  Level-2 M-file S-Function/2 -> Out2/1
  Level-2 M-file S-Function/3 -> Out3/1
  Level-2 M-file S-Function/5 -> Out5/1
  Level-2 M-file S-Function/6 -> Out6/1
  Level-2 M-file S-Function/4 -> Out4/1
  Level-2 M-file S-Function/1 -> Out1/1
  Level-2 M-file S-Function/10 -> Out10/1
  Level-2 M-file S-Function/9 -> Out9/1
  Level-2 M-file S-Function/8 -> Out8/1
  Level-2 M-file S-Function/7 -> Out7/1

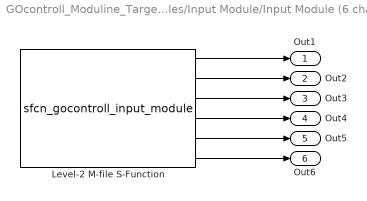
== system GOcontroll_Moduline_Target/Modules/Input Module/Input Module (6 channel) ==
  Level-2 M-file S-Function : M-S-Function  FunctionName=sfcn_gocontroll_input_module  Parameters=tsamp, moduleSlot,ContrType,C1func,C1volt,C1afil,C1dpul,C1pu,C1pd,C2func,C2volt,C2afil,C2dpul,C2pu,C2pd,C3func,C3volt,C3afil,C3dpul,C3pu,C3pd,C4func,C4volt,C4afil,C4dpul,C4pu,C4pd,C5func,C5volt,C5afil,C5dpul,C5pu,C5pd,C6func,C6volt,C6afil,C6dpul,C6pu,C6pd,SensSup1,SensSup2,SensSup3
  Out1 : Outport
  Out2 : Outport  Port=2
  Out3 : Outport  Port=3
  Out4 : Outport  Port=4
  Out5 : Outport  Port=5
  Out6 : Outport  Port=6
  wires:
  Level-2 M-file S-Function/2 -> Out2/1
  Level-2 M-file S-Function/3 -> Out3/1
  Level-2 M-file S-Function/5 -> Out5/1
  Level-2 M-file S-Function/6 -> Out6/1
  Level-2 M-file S-Function/4 -> Out4/1
  Level-2 M-file S-Function/1 -> Out1/1

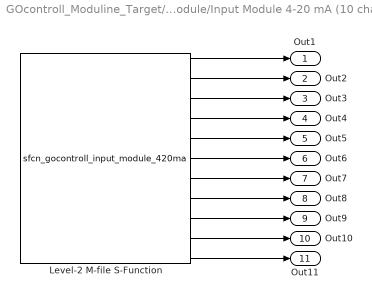
== system GOcontroll_Moduline_Target/Modules/Input Module/Input Module 4-20 mA (10 channel) ==
  Level-2 M-file S-Function : M-S-Function  FunctionName=sfcn_gocontroll_input_module_420ma  Parameters=tsamp, moduleSlot,Sup16va
  Out1 : Outport
  Out2 : Outport  Port=2
  Out3 : Outport  Port=3
  Out4 : Outport  Port=4
  Out5 : Outport  Port=5
  Out6 : Outport  Port=6
  Out7 : Outport  Port=7
  Out8 : Outport  Port=8
  Out9 : Outport  Port=9
  Out10 : Outport  Port=10
  Out11 : Outport  Port=11
  wires:
  Level-2 M-file S-Function/2 -> Out2/1
  Level-2 M-file S-Function/3 -> Out3/1
  Level-2 M-file S-Function/5 -> Out5/1
  Level-2 M-file S-Function/6 -> Out6/1
  Level-2 M-file S-Function/4 -> Out4/1
  Level-2 M-file S-Function/1 -> Out1/1
  Level-2 M-file S-Function/10 -> Out10/1
  Level-2 M-file S-Function/9 -> Out9/1
  Level-2 M-file S-Function/8 -> Out8/1
  Level-2 M-file S-Function/7 -> Out7/1
  Level-2 M-file S-Function/11 -> Out11/1

== system GOcontroll_Moduline_Target/Modules/Input Module/Reset Puls Counter (6 channel) ==
  In1 : Inport
  In2 : Inport  Port=2
  Level-2 M-file S-Function : M-S-Function  FunctionName=sfcn_gocontroll_input_module_reset  Parameters=tsamp, moduleSlot,contrType,channel
  wires:
  In2/1 -> Level-2 M-file S-Function/2
  In1/1 -> Level-2 M-file S-Function/1

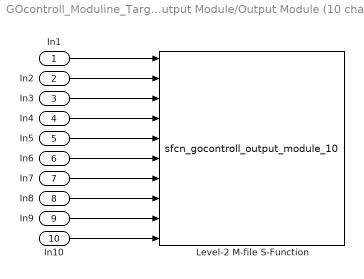
== system GOcontroll_Moduline_Target/Modules/Output Module/Output Module (10 channel) ==
  In1 : Inport
  In2 : Inport  Port=2
  In3 : Inport  Port=3
  In4 : Inport  Port=4
  In5 : Inport  Port=5
  In6 : Inport  Port=6
  In7 : Inport  Port=7
  In8 : Inport  Port=8
  In9 : Inport  Port=9
  In10 : Inport  Port=10
  Level-2 M-file S-Function : M-S-Function  FunctionName=sfcn_gocontroll_output_module_10  Parameters=tsamp, moduleSlot,C12freq,C1func,C2func,C34freq,C3func,C4func,C56freq,C5func,C6func,C78freq,C7func,C8func,C910freq,C9func,C10func,C1peakDuty,C1peakTime,C2peakDuty,C2peakTime,C3peakDuty,C3peakTime,C4peakDuty,C4peakTime,C5peakDuty,C5peakTime,C6peakDuty,C6peakTime,C7peakDuty,C7peakTime,C8peakDuty,C8peakTime,C9peakDuty,C9peakTime,C10peakDuty,C10peakTime
  wires:
  In3/1 -> Level-2 M-file S-Function/3
  In6/1 -> Level-2 M-file S-Function/6
  In5/1 -> Level-2 M-file S-Function/5
  In4/1 -> Level-2 M-file S-Function/4
  In2/1 -> Level-2 M-file S-Function/2
  In1/1 -> Level-2 M-file S-Function/1
  In9/1 -> Level-2 M-file S-Function/9
  In10/1 -> Level-2 M-file S-Function/10
  In7/1 -> Level-2 M-file S-Function/7
  In8/1 -> Level-2 M-file S-Function/8

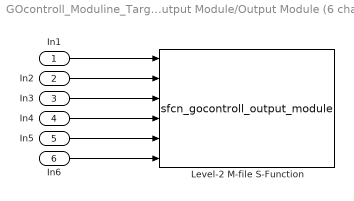
== system GOcontroll_Moduline_Target/Modules/Output Module/Output Module (6 channel) ==
  In1 : Inport
  In2 : Inport  Port=2
  In3 : Inport  Port=3
  In4 : Inport  Port=4
  In5 : Inport  Port=5
  In6 : Inport  Port=6
  Level-2 M-file S-Function : M-S-Function  FunctionName=sfcn_gocontroll_output_module  Parameters=tsamp, moduleSlot,ContrType,C12freq,C1func,C2func,C34freq,C3func,C4func,C56freq,C5func,C6func,C1cur,C2cur,C3cur,C4cur,C5cur,C6cur,C1peakCurrent,C1peakTime,C2peakCurrent,C2peakTime,C3peakCurrent,C3peakTime,C4peakCurrent,C4peakTime,C5peakCurrent,C5peakTime,C6peakCurrent,C6peakTime
  wires:
  In3/1 -> Level-2 M-file S-Function/3
  In6/1 -> Level-2 M-file S-Function/6
  In5/1 -> Level-2 M-file S-Function/5
  In4/1 -> Level-2 M-file S-Function/4
  In2/1 -> Level-2 M-file S-Function/2
  In1/1 -> Level-2 M-file S-Function/1

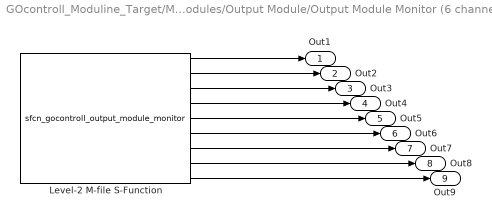
== system GOcontroll_Moduline_Target/Modules/Output Module/Output Module Monitor (6 channel) ==
  Level-2 M-file S-Function : M-S-Function  FunctionName=sfcn_gocontroll_output_module_monitor  Parameters=tsamp, moduleSlot, ContrType
  Out1 : Outport
  Out2 : Outport  Port=2
  Out3 : Outport  Port=3
  Out4 : Outport  Port=4
  Out5 : Outport  Port=5
  Out6 : Outport  Port=6
  Out7 : Outport  Port=7
  Out8 : Outport  Port=8
  Out9 : Outport  Port=9
  wires:
  Level-2 M-file S-Function/8 -> Out8/1
  Level-2 M-file S-Function/1 -> Out1/1
  Level-2 M-file S-Function/2 -> Out2/1
  Level-2 M-file S-Function/3 -> Out3/1
  Level-2 M-file S-Function/4 -> Out4/1
  Level-2 M-file S-Function/5 -> Out5/1
  Level-2 M-file S-Function/6 -> Out6/1
  Level-2 M-file S-Function/7 -> Out7/1
  Level-2 M-file S-Function/9 -> Out9/1

== system GOcontroll_Moduline_Target/Network/UDP/Configure UDP socket ==
  Level-2 MATLAB S-Function : M-S-Function  FunctionName=sfcn_UDPConfig  Parameters=tsamp, port, ip, broadcast

== system GOcontroll_Moduline_Target/Network/UDP/UDP Send old ==
  Message : Inport
  Constant : Constant  Value=0  OutDataTypeStr=uint8
  Gnd : Ground
  Level-2 MATLAB S-Function : M-S-Function  FunctionName=sfcn_UDPSend  Parameters=tsamp,port,ip,id,input_type
  Vector Concatenate : Concatenate
  wires:
  Vector Concatenate/1 -> Level-2 MATLAB S-Function/2
  Message/1 -> Vector Concatenate/2
  Constant/1 -> Vector Concatenate/1
  Gnd/1 -> Level-2 MATLAB S-Function/1

== system GOcontroll_Moduline_Target/Network/UDP/UDP receive old ==
  Gnd : Ground
  Level-2 MATLAB S-Function1 : M-S-Function  FunctionName=sfcn_UDPReceive  Parameters=tsamp,id,buff_len,input_type
  Selector : Selector  IndexMode=Zero-based  InputPortWidth=buff_len+1  IndexOptions=Starting index (dialog)  Indices=[1]  OutputSizes=buff_len
  newMessage : Outport
  Message : Outport  Port=2
  wires:
  Level-2 MATLAB S-Function1/1 -> newMessage/1
  Level-2 MATLAB S-Function1/2 -> Selector/1
  Selector/1 -> Message/1
  Gnd/1 -> Level-2 MATLAB S-Function1/1

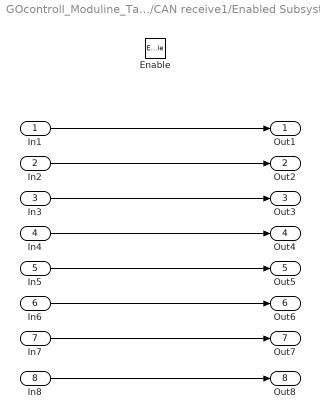
== system GOcontroll_Moduline_Target/CAN/CAN 2.0B/CAN receive1/Enabled Subsystem ==
  In1 : Inport
  In2 : Inport  Port=2
  In3 : Inport  Port=3
  In4 : Inport  Port=4
  In5 : Inport  Port=5
  In6 : Inport  Port=6
  In7 : Inport  Port=7
  In8 : Inport  Port=8
  Enable : EnablePort
  Out1 : Outport
  Out2 : Outport  Port=2
  Out3 : Outport  Port=3
  Out4 : Outport  Port=4
  Out5 : Outport  Port=5
  Out6 : Outport  Port=6
  Out7 : Outport  Port=7
  Out8 : Outport  Port=8
  wires:
  In1/1 -> Out1/1
  In2/1 -> Out2/1
  In3/1 -> Out3/1
  In4/1 -> Out4/1
  In5/1 -> Out5/1
  In6/1 -> Out6/1
  In7/1 -> Out7/1
  In8/1 -> Out8/1
